simulink model "ultima"  (R2016a)
settings: Solver=ode45  SolverMode=SingleTasking  StartTime=0.0  StopTime=5/60  RelTol=1e-3
libraries: powerlib x98, powerlib_meascontrol x14
settings Model: Creator=hiago  LastModifiedBy=hiago
settings DebuggingCC: SFUnexpectedBacktrackingDiag=error  SFNoUnconditionalDefaultTransitionDiag=error
settings SFSimCC: SimUseLocalCustomCode=on
settings RTWCC: RTWUseLocalCustomCode=on
settings GRTTargetCC: TargetLangStandard=C99 (ISO)  GeneratePreprocessorConditionals=Use local settings
settings ConfigComp: CovMetricSettings=dwe  CovHtmlReporting=off  CovSaveCumulativeToWorkspaceVar=off  CovSaveSingleToWorkspaceVar=off  CovExternalEMLEnable=on

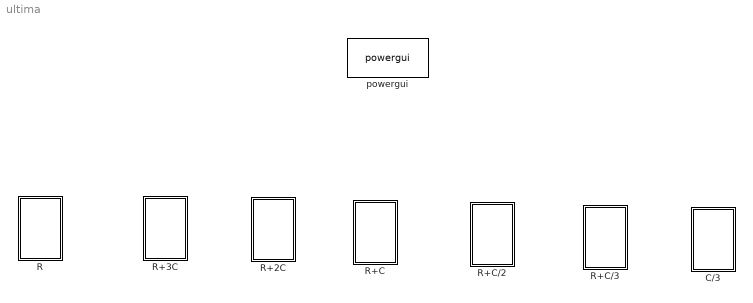
== system ultima ==
  C/3 : Subsystem
  R : Subsystem
  R+2C : Subsystem
  R+3C : Subsystem
  R+C : Subsystem
  R+C/2 : Subsystem
  R+C/3 : Subsystem
  powergui : powerlib/powergui  Priority=1  SimulationMode=Discrete  SampleTime=5e-5  frequency=60  Iterations=50  frequencyindice=60  Pbase=100e6  ErrMax=1e-4  UnitsV=kV  UnitsW=MW  buscounter=0  FunctionMessages=off  echomessages=off  EnableUseOfTLC=off  CurrentSourceSwitches=off  DisableSnubberDevices=off  DisableRonSwitches=off  DisableVfSwitches=off  DisplayEquations=off  SolverType=Tustin/Backward Euler (TBE)  Interpol=off  ExternalGateDelay=off  methode=off  Ts=100  x0status=blocks  SPID=on  SwTol=0  HookPort=off  RestoreLinks=warning  ResistiveCurrentMeasurement=off  Frange=[0:2:500]  Ylog=off  Xlog=on  ShowGrid=off  save=off  variable=ZData  structure=0  ZoomFFT=off  StartTime=0.0  cycles=1  DisplayStyle=1  fundamental=60  FreqAxis=off  MaxFrequency=1000  frequencyindicesteady=1  RmsSteady=1  display=off

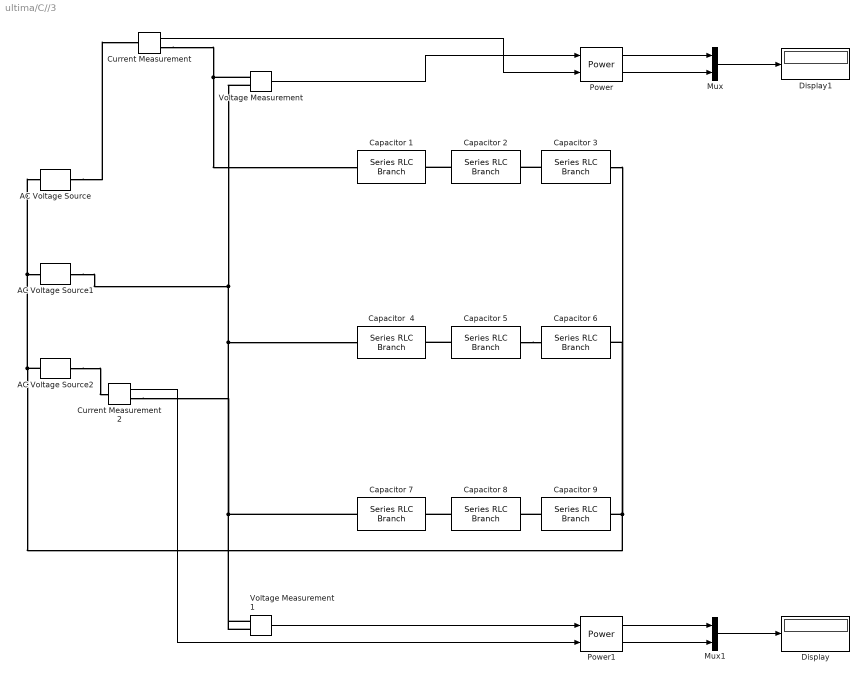
== system ultima/C//3 ==
  AC Voltage Source : powerlib/Electrical Sources/AC Voltage Source  Amplitude=127*sqrt(2)  Phase=0  Frequency=60  SampleTime=5e-5  Measurements=None  BusType=swing  Pref=10e3  Qref=0  Qmin=-inf  Qmax=+inf
  AC Voltage Source1 : powerlib/Electrical Sources/AC Voltage Source  Amplitude=127*sqrt(2)  Phase=-120  Frequency=60  SampleTime=5e-5  Measurements=None  BusType=swing  Pref=10e3  Qref=0  Qmin=-inf  Qmax=+inf
  AC Voltage Source2 : powerlib/Electrical Sources/AC Voltage Source  Amplitude=127*sqrt(2)  Phase=120  Frequency=60  SampleTime=5e-5  Measurements=None  BusType=swing  Pref=10e3  Qref=0  Qmin=-inf  Qmax=+inf
  Capacitor  4 : powerlib/Elements/Series RLC Branch  LConnTagsString=__new0  RConnTagsString=__new0  BranchType=RC  Resistance=1  Inductance=1e-3  SetiL0=off  InitialCurrent=0  Capacitance=22e-6  Setx0=off  InitialVoltage=0  Measurements=None
  "Capacitor 1 " : powerlib/Elements/Series RLC Branch  LConnTagsString=__new0  RConnTagsString=__new0  BranchType=RC  Resistance=1  Inductance=1e-3  SetiL0=off  InitialCurrent=0  Capacitance=22e-6  Setx0=off  InitialVoltage=0  Measurements=None
  Capacitor {2..3,6,8..9} (5 alike) : powerlib/Elements/Series RLC Branch  LConnTagsString=__new0  RConnTagsString=__new0  BranchType=C  Resistance=100  Inductance=1e-3  SetiL0=off  InitialCurrent=0  Capacitance=22e-6  Setx0=off  InitialVoltage=0  Measurements=None
  "Capacitor 5 " : powerlib/Elements/Series RLC Branch  LConnTagsString=__new0  RConnTagsString=__new0  BranchType=C  Resistance=100  Inductance=1e-3  SetiL0=off  InitialCurrent=0  Capacitance=22e-6  Setx0=off  InitialVoltage=0  Measurements=None
  Capacitor 7 : powerlib/Elements/Series RLC Branch  LConnTagsString=__new0  RConnTagsString=__new0  BranchType=RC  Resistance=1  Inductance=1e-3  SetiL0=off  InitialCurrent=0  Capacitance=22e-6  Setx0=off  InitialVoltage=0  Measurements=None
  Current Measurement : powerlib/Measurements/Current Measurement  PhasorSimulation=off  OutputType=Complex  PSBequivalent=0
  Current Measurement2 : powerlib/Measurements/Current Measurement  PhasorSimulation=off  OutputType=Complex  PSBequivalent=0
  Display : Display
  Display1 : Display
  Mux : Mux  Inputs=2
  Mux1 : Mux  Inputs=2
  Power : powerlib_meascontrol/Measurements/Power  Freq=60  Vinit=[1, 0]  Iinit=[1, 0]  Ts=5e-5
  Power1 : powerlib_meascontrol/Measurements/Power  Freq=60  Vinit=[1, 0]  Iinit=[1, 0]  Ts=5e-5
  Voltage Measurement : powerlib/Measurements/Voltage Measurement  PhasorSimulation=off  OutputType=Complex  PSBequivalent=0
  Voltage Measurement1 : powerlib/Measurements/Voltage Measurement  PhasorSimulation=off  OutputType=Complex  PSBequivalent=0
  wires:
  Power1/2 -> Mux1/2
  Power/2 -> Mux/2
  Current Measurement2/1 -> Power1/2
  Current Measurement/1 -> Power/2
  Voltage Measurement/1 -> Power/1
  Power/1 -> Mux/1
  Mux/1 -> Display1/1
  Power1/1 -> Mux1/1
  Voltage Measurement1/1 -> Power1/1
  Mux1/1 -> Display/1
  connections:
  AC Voltage Source2/LConn1 -- Capacitor 6/LConn1 -- Capacitor 3/LConn1 -- Capacitor 9/LConn1 -- AC Voltage Source/LConn1 -- AC Voltage Source1/LConn1
  Voltage Measurement1/LConn1 -- Capacitor 7/RConn1 -- Current Measurement2/RConn1
  AC Voltage Source/RConn1 -- Current Measurement/LConn1
  Current Measurement/RConn1 -- "Capacitor 1 "/RConn1 -- Voltage Measurement/LConn1
  Capacitor 2/RConn1 -- "Capacitor 1 "/LConn1
  AC Voltage Source2/RConn1 -- Current Measurement2/LConn1
  Voltage Measurement1/LConn2 -- Capacitor  4/RConn1 -- AC Voltage Source1/RConn1 -- Voltage Measurement/LConn2
  Capacitor 3/RConn1 -- Capacitor 2/LConn1
  "Capacitor 5 "/RConn1 -- Capacitor  4/LConn1
  "Capacitor 5 "/LConn1 -- Capacitor 6/RConn1
  Capacitor 9/RConn1 -- Capacitor 8/LConn1
  Capacitor 8/RConn1 -- Capacitor 7/LConn1

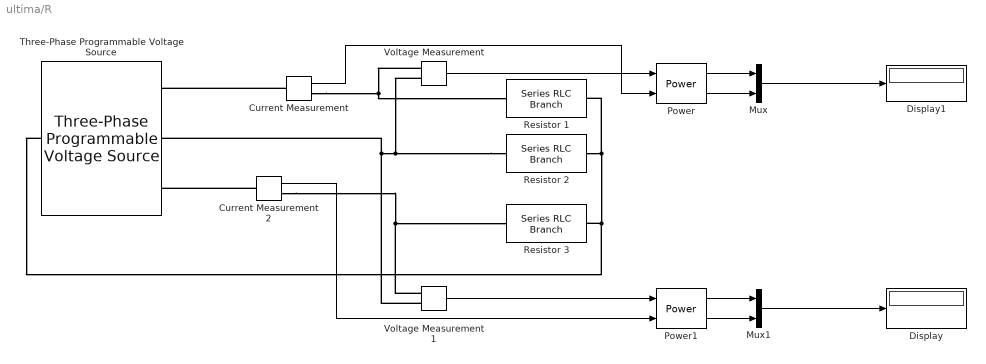
== system ultima/R ==
  Current Measurement : powerlib/Measurements/Current Measurement  PhasorSimulation=off  OutputType=Complex  PSBequivalent=0
  Current Measurement2 : powerlib/Measurements/Current Measurement  PhasorSimulation=off  OutputType=Complex  PSBequivalent=0
  Display : Display
  Display1 : Display
  Mux : Mux  Inputs=2
  Mux1 : Mux  Inputs=2
  Power : powerlib_meascontrol/Measurements/Power  Freq=60  Vinit=[1, 0]  Iinit=[1, 0]  Ts=5e-5
  Power1 : powerlib_meascontrol/Measurements/Power  Freq=60  Vinit=[1, 0]  Iinit=[1, 0]  Ts=5e-5
  Resistor 1 : powerlib/Elements/Series RLC Branch  LConnTagsString=__new0  RConnTagsString=__new0  BranchType=R  Resistance=100  Inductance=1e-3  SetiL0=off  InitialCurrent=0  Capacitance=1e-6  Setx0=off  InitialVoltage=0  Measurements=None
  Resistor 2 : powerlib/Elements/Series RLC Branch  LConnTagsString=__new0  RConnTagsString=__new0  BranchType=R  Resistance=100  Inductance=1e-3  SetiL0=off  InitialCurrent=0  Capacitance=1e-6  Setx0=off  InitialVoltage=0  Measurements=None
  Resistor 3 : powerlib/Elements/Series RLC Branch  LConnTagsString=__new0  RConnTagsString=__new0  BranchType=R  Resistance=100  Inductance=1e-3  SetiL0=off  InitialCurrent=0  Capacitance=1e-6  Setx0=off  InitialVoltage=0  Measurements=None
  Three-Phase Programmable Voltage Source : powerlib/Electrical Sources/Three-Phase Programmable Voltage Source  PositiveSequence="[220  0 60]"  VariationEntity=None  VariationType=Table of time-amplitude pairs  VariationTypeAlt=Step  VariationStep=0.5  VariationRate=10  VariationMagnitude=0.3  VariationFrequency=2  VariationTiming=[1 2]  VariationPhaseA=off  Amplitudes=[1 0.8 1.2 1.0]  TimeValues=[0 0.1 0.15 0.2]  HarmonicGeneration=off  HarmonicA=[3 0.2 -25 0]  HarmonicB=[2 0.15 35 2]  Timing="[0.05  3]"  BusType=swing  Pref=0  Qref=0  Qmin=-inf  Qmax=inf
  Voltage Measurement : powerlib/Measurements/Voltage Measurement  PhasorSimulation=off  OutputType=Complex  PSBequivalent=0
  Voltage Measurement1 : powerlib/Measurements/Voltage Measurement  PhasorSimulation=off  OutputType=Complex  PSBequivalent=0
  wires:
  Mux1/1 -> Display/1
  Voltage Measurement1/1 -> Power1/1
  Voltage Measurement/1 -> Power/1
  Power1/2 -> Mux1/2
  Current Measurement/1 -> Power/2
  Power/1 -> Mux/1
  Mux/1 -> Display1/1
  Power/2 -> Mux/2
  Power1/1 -> Mux1/1
  Current Measurement2/1 -> Power1/2
  connections:
  Voltage Measurement1/LConn1 -- Resistor 3/LConn1 -- Current Measurement2/RConn1
  Current Measurement/RConn1 -- Resistor 1/LConn1 -- Voltage Measurement/LConn1
  Current Measurement/LConn1 -- Three-Phase Programmable Voltage Source/RConn1
  Resistor 2/LConn1 -- Voltage Measurement1/LConn2 -- Three-Phase Programmable Voltage Source/RConn2 -- Voltage Measurement/LConn2
  Resistor 2/RConn1 -- Three-Phase Programmable Voltage Source/LConn1 -- Resistor 3/RConn1 -- Resistor 1/RConn1
  Current Measurement2/LConn1 -- Three-Phase Programmable Voltage Source/RConn3

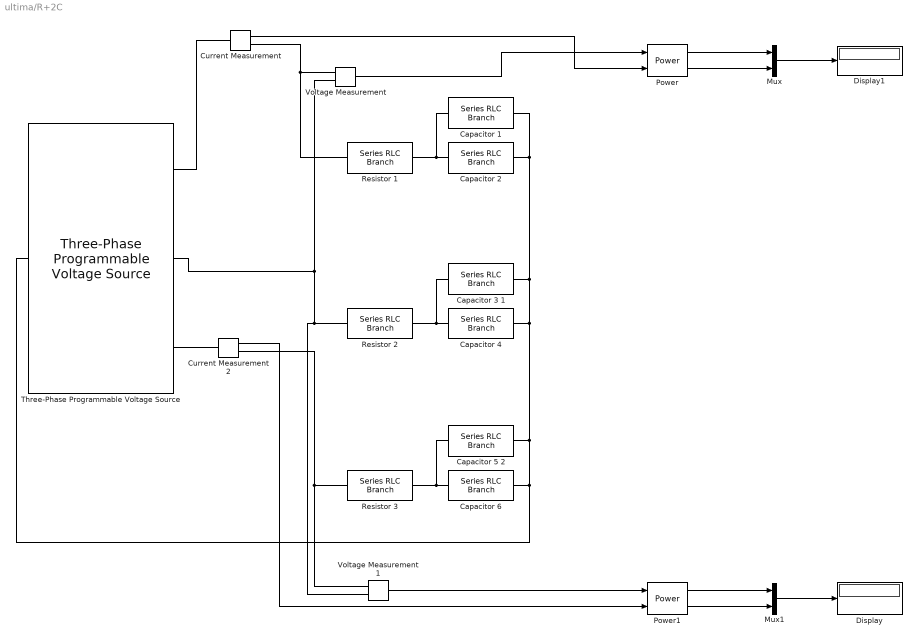
== system ultima/R+2C ==
  "Capacitor 1 " : powerlib/Elements/Series RLC Branch  LConnTagsString=__new0  RConnTagsString=__new0  BranchType=C  Resistance=100  Inductance=1e-3  SetiL0=off  InitialCurrent=0  Capacitance=22e-6  Setx0=off  InitialVoltage=0  Measurements=None
  Capacitor 2 : powerlib/Elements/Series RLC Branch  LConnTagsString=__new0  RConnTagsString=__new0  BranchType=C  Resistance=100  Inductance=1e-3  SetiL0=off  InitialCurrent=0  Capacitance=22e-6  Setx0=off  InitialVoltage=0  Measurements=None
  Capacitor 3 1 : powerlib/Elements/Series RLC Branch  LConnTagsString=__new0  RConnTagsString=__new0  BranchType=C  Resistance=100  Inductance=1e-3  SetiL0=off  InitialCurrent=0  Capacitance=22e-6  Setx0=off  InitialVoltage=0  Measurements=None
  Capacitor 4 : powerlib/Elements/Series RLC Branch  LConnTagsString=__new0  RConnTagsString=__new0  BranchType=C  Resistance=100  Inductance=1e-3  SetiL0=off  InitialCurrent=0  Capacitance=22e-6  Setx0=off  InitialVoltage=0  Measurements=None
  Capacitor 5 2 : powerlib/Elements/Series RLC Branch  LConnTagsString=__new0  RConnTagsString=__new0  BranchType=C  Resistance=100  Inductance=1e-3  SetiL0=off  InitialCurrent=0  Capacitance=22e-6  Setx0=off  InitialVoltage=0  Measurements=None
  Capacitor 6 : powerlib/Elements/Series RLC Branch  LConnTagsString=__new0  RConnTagsString=__new0  BranchType=C  Resistance=100  Inductance=1e-3  SetiL0=off  InitialCurrent=0  Capacitance=22e-6  Setx0=off  InitialVoltage=0  Measurements=None
  Current Measurement : powerlib/Measurements/Current Measurement  PhasorSimulation=off  OutputType=Complex  PSBequivalent=0
  Current Measurement2 : powerlib/Measurements/Current Measurement  PhasorSimulation=off  OutputType=Complex  PSBequivalent=0
  Display : Display
  Display1 : Display
  Mux : Mux  Inputs=2
  Mux1 : Mux  Inputs=2
  Power : powerlib_meascontrol/Measurements/Power  Freq=60  Vinit=[1, 0]  Iinit=[1, 0]  Ts=5e-5
  Power1 : powerlib_meascontrol/Measurements/Power  Freq=60  Vinit=[1, 0]  Iinit=[1, 0]  Ts=5e-5
  Resistor 1 : powerlib/Elements/Series RLC Branch  LConnTagsString=__new0  RConnTagsString=__new0  BranchType=R  Resistance=100  Inductance=1e-3  SetiL0=off  InitialCurrent=0  Capacitance=1e-6  Setx0=off  InitialVoltage=0  Measurements=None
  Resistor 2 : powerlib/Elements/Series RLC Branch  LConnTagsString=__new0  RConnTagsString=__new0  BranchType=R  Resistance=100  Inductance=1e-3  SetiL0=off  InitialCurrent=0  Capacitance=1e-6  Setx0=off  InitialVoltage=0  Measurements=None
  Resistor 3 : powerlib/Elements/Series RLC Branch  LConnTagsString=__new0  RConnTagsString=__new0  BranchType=R  Resistance=100  Inductance=1e-3  SetiL0=off  InitialCurrent=0  Capacitance=1e-6  Setx0=off  InitialVoltage=0  Measurements=None
  Three-Phase Programmable Voltage Source : powerlib/Electrical Sources/Three-Phase Programmable Voltage Source  PositiveSequence="[220  0 60]"  VariationEntity=None  VariationType=Table of time-amplitude pairs  VariationTypeAlt=Step  VariationStep=0.5  VariationRate=10  VariationMagnitude=0.3  VariationFrequency=2  VariationTiming=[1 2]  VariationPhaseA=off  Amplitudes=[1 0.8 1.2 1.0]  TimeValues=[0 0.1 0.15 0.2]  HarmonicGeneration=off  HarmonicA=[3 0.2 -25 0]  HarmonicB=[2 0.15 35 2]  Timing="[0.05  3]"  BusType=swing  Pref=0  Qref=0  Qmin=-inf  Qmax=inf
  Voltage Measurement : powerlib/Measurements/Voltage Measurement  PhasorSimulation=off  OutputType=Complex  PSBequivalent=0
  Voltage Measurement1 : powerlib/Measurements/Voltage Measurement  PhasorSimulation=off  OutputType=Complex  PSBequivalent=0
  wires:
  Voltage Measurement1/1 -> Power1/1
  Power1/2 -> Mux1/2
  Power/1 -> Mux/1
  Power1/1 -> Mux1/1
  Mux1/1 -> Display/1
  Current Measurement2/1 -> Power1/2
  Power/2 -> Mux/2
  Voltage Measurement/1 -> Power/1
  Current Measurement/1 -> Power/2
  Mux/1 -> Display1/1
  connections:
  Resistor 3/LConn1 -- Current Measurement2/RConn1 -- Voltage Measurement1/LConn1
  Current Measurement/RConn1 -- Resistor 1/LConn1 -- Voltage Measurement/LConn1
  Voltage Measurement/LConn2 -- Voltage Measurement1/LConn2 -- Resistor 2/LConn1 -- Three-Phase Programmable Voltage Source/RConn2
  Current Measurement/LConn1 -- Three-Phase Programmable Voltage Source/RConn1
  Current Measurement2/LConn1 -- Three-Phase Programmable Voltage Source/RConn3
  Capacitor 6/RConn1 -- Three-Phase Programmable Voltage Source/LConn1 -- Capacitor 5 2/RConn1 -- Capacitor 4/RConn1 -- Capacitor 3 1/RConn1 -- Capacitor 2/RConn1 -- "Capacitor 1 "/RConn1
  Capacitor 5 2/LConn1 -- Resistor 3/RConn1 -- Capacitor 6/LConn1
  Capacitor 4/LConn1 -- Resistor 2/RConn1 -- Capacitor 3 1/LConn1
  Capacitor 2/LConn1 -- Resistor 1/RConn1 -- "Capacitor 1 "/LConn1

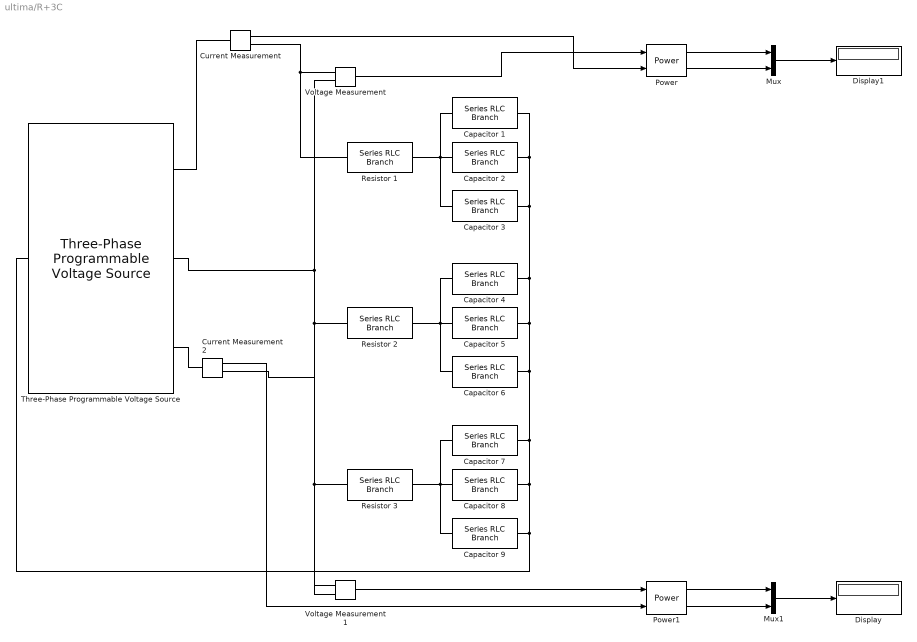
== system ultima/R+3C ==
  Capacitor {1..9} (9 alike) : powerlib/Elements/Series RLC Branch  LConnTagsString=__new0  RConnTagsString=__new0  BranchType=C  Resistance=100  Inductance=1e-3  SetiL0=off  InitialCurrent=0  Capacitance=22e-6  Setx0=off  InitialVoltage=0  Measurements=None
  Current Measurement : powerlib/Measurements/Current Measurement  PhasorSimulation=off  OutputType=Complex  PSBequivalent=0
  Current Measurement2 : powerlib/Measurements/Current Measurement  PhasorSimulation=off  OutputType=Complex  PSBequivalent=0
  Display : Display
  Display1 : Display
  Mux : Mux  Inputs=2
  Mux1 : Mux  Inputs=2
  Power : powerlib_meascontrol/Measurements/Power  Freq=60  Vinit=[1, 0]  Iinit=[1, 0]  Ts=5e-5
  Power1 : powerlib_meascontrol/Measurements/Power  Freq=60  Vinit=[1, 0]  Iinit=[1, 0]  Ts=5e-5
  Resistor 1 : powerlib/Elements/Series RLC Branch  LConnTagsString=__new0  RConnTagsString=__new0  BranchType=R  Resistance=100  Inductance=1e-3  SetiL0=off  InitialCurrent=0  Capacitance=1e-6  Setx0=off  InitialVoltage=0  Measurements=None
  Resistor 2 : powerlib/Elements/Series RLC Branch  LConnTagsString=__new0  RConnTagsString=__new0  BranchType=R  Resistance=100  Inductance=1e-3  SetiL0=off  InitialCurrent=0  Capacitance=1e-6  Setx0=off  InitialVoltage=0  Measurements=None
  Resistor 3 : powerlib/Elements/Series RLC Branch  LConnTagsString=__new0  RConnTagsString=__new0  BranchType=R  Resistance=100  Inductance=1e-3  SetiL0=off  InitialCurrent=0  Capacitance=1e-6  Setx0=off  InitialVoltage=0  Measurements=None
  Three-Phase Programmable Voltage Source : powerlib/Electrical Sources/Three-Phase Programmable Voltage Source  PositiveSequence="[220  0 60]"  VariationEntity=None  VariationType=Table of time-amplitude pairs  VariationTypeAlt=Step  VariationStep=0.5  VariationRate=10  VariationMagnitude=0.3  VariationFrequency=2  VariationTiming=[1 2]  VariationPhaseA=off  Amplitudes=[1 0.8 1.2 1.0]  TimeValues=[0 0.1 0.15 0.2]  HarmonicGeneration=off  HarmonicA=[3 0.2 -25 0]  HarmonicB=[2 0.15 35 2]  Timing="[0.05  3]"  BusType=swing  Pref=0  Qref=0  Qmin=-inf  Qmax=inf
  Voltage Measurement : powerlib/Measurements/Voltage Measurement  PhasorSimulation=off  OutputType=Complex  PSBequivalent=0
  Voltage Measurement1 : powerlib/Measurements/Voltage Measurement  PhasorSimulation=off  OutputType=Complex  PSBequivalent=0
  wires:
  Current Measurement/1 -> Power/2
  Power1/1 -> Mux1/1
  Current Measurement2/1 -> Power1/2
  Power/1 -> Mux/1
  Voltage Measurement/1 -> Power/1
  Mux/1 -> Display1/1
  Power/2 -> Mux/2
  Mux1/1 -> Display/1
  Voltage Measurement1/1 -> Power1/1
  Power1/2 -> Mux1/2
  connections:
  Current Measurement2/LConn1 -- Three-Phase Programmable Voltage Source/RConn3
  Current Measurement2/RConn1 -- Voltage Measurement1/LConn1 -- Resistor 3/LConn1
  Current Measurement/RConn1 -- Resistor 1/LConn1 -- Voltage Measurement/LConn1
  Resistor 2/LConn1 -- Three-Phase Programmable Voltage Source/RConn2 -- Voltage Measurement/LConn2 -- Voltage Measurement1/LConn2
  Current Measurement/LConn1 -- Three-Phase Programmable Voltage Source/RConn1
  Capacitor 3/LConn1 -- Capacitor 1/LConn1 -- Resistor 1/RConn1 -- Capacitor 2/LConn1
  Capacitor 8/RConn1 -- Three-Phase Programmable Voltage Source/LConn1 -- Capacitor 9/RConn1 -- Capacitor 5/RConn1 -- Capacitor 1/RConn1 -- Capacitor 2/RConn1 -- Capacitor 3/RConn1 -- Capacitor 4/RConn1 -- Capacitor 6/RConn1 -- Capacitor 7/RConn1
  Resistor 2/RConn1 -- Capacitor 6/LConn1 -- Capacitor 4/LConn1 -- Capacitor 5/LConn1
  Capacitor 8/LConn1 -- Capacitor 9/LConn1 -- Resistor 3/RConn1 -- Capacitor 7/LConn1

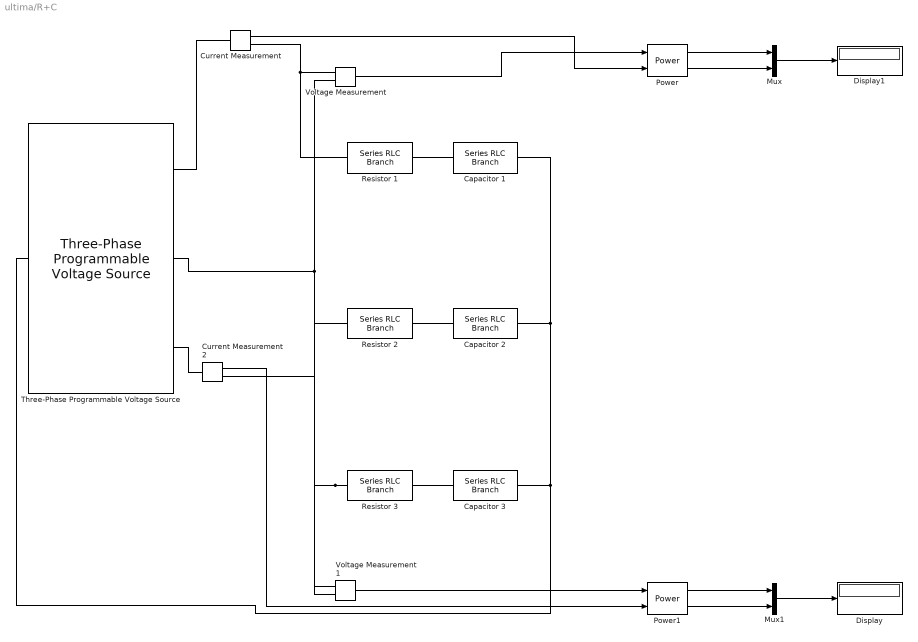
== system ultima/R+C ==
  Capacitor 1 : powerlib/Elements/Series RLC Branch  LConnTagsString=__new0  RConnTagsString=__new0  BranchType=C  Resistance=100  Inductance=1e-3  SetiL0=off  InitialCurrent=0  Capacitance=22e-6  Setx0=off  InitialVoltage=0  Measurements=None
  Capacitor 2 : powerlib/Elements/Series RLC Branch  LConnTagsString=__new0  RConnTagsString=__new0  BranchType=C  Resistance=100  Inductance=1e-3  SetiL0=off  InitialCurrent=0  Capacitance=22e-6  Setx0=off  InitialVoltage=0  Measurements=None
  Capacitor 3 : powerlib/Elements/Series RLC Branch  LConnTagsString=__new0  RConnTagsString=__new0  BranchType=C  Resistance=100  Inductance=1e-3  SetiL0=off  InitialCurrent=0  Capacitance=22e-6  Setx0=off  InitialVoltage=0  Measurements=None
  Current Measurement : powerlib/Measurements/Current Measurement  PhasorSimulation=off  OutputType=Complex  PSBequivalent=0
  Current Measurement2 : powerlib/Measurements/Current Measurement  PhasorSimulation=off  OutputType=Complex  PSBequivalent=0
  Display : Display
  Display1 : Display
  Mux : Mux  Inputs=2
  Mux1 : Mux  Inputs=2
  Power : powerlib_meascontrol/Measurements/Power  Freq=60  Vinit=[1, 0]  Iinit=[1, 0]  Ts=5e-5
  Power1 : powerlib_meascontrol/Measurements/Power  Freq=60  Vinit=[1, 0]  Iinit=[1, 0]  Ts=5e-5
  Resistor 1 : powerlib/Elements/Series RLC Branch  LConnTagsString=__new0  RConnTagsString=__new0  BranchType=R  Resistance=100  Inductance=1e-3  SetiL0=off  InitialCurrent=0  Capacitance=1e-6  Setx0=off  InitialVoltage=0  Measurements=None
  Resistor 2 : powerlib/Elements/Series RLC Branch  LConnTagsString=__new0  RConnTagsString=__new0  BranchType=R  Resistance=100  Inductance=1e-3  SetiL0=off  InitialCurrent=0  Capacitance=1e-6  Setx0=off  InitialVoltage=0  Measurements=None
  Resistor 3 : powerlib/Elements/Series RLC Branch  LConnTagsString=__new0  RConnTagsString=__new0  BranchType=R  Resistance=100  Inductance=1e-3  SetiL0=off  InitialCurrent=0  Capacitance=1e-6  Setx0=off  InitialVoltage=0  Measurements=None
  Three-Phase Programmable Voltage Source : powerlib/Electrical Sources/Three-Phase Programmable Voltage Source  PositiveSequence="[220  0 60]"  VariationEntity=None  VariationType=Table of time-amplitude pairs  VariationTypeAlt=Step  VariationStep=0.5  VariationRate=10  VariationMagnitude=0.3  VariationFrequency=2  VariationTiming=[1 2]  VariationPhaseA=off  Amplitudes=[1 0.8 1.2 1.0]  TimeValues=[0 0.1 0.15 0.2]  HarmonicGeneration=off  HarmonicA=[3 0.2 -25 0]  HarmonicB=[2 0.15 35 2]  Timing="[0.05  3]"  BusType=swing  Pref=0  Qref=0  Qmin=-inf  Qmax=inf
  Voltage Measurement : powerlib/Measurements/Voltage Measurement  PhasorSimulation=off  OutputType=Complex  PSBequivalent=0
  Voltage Measurement1 : powerlib/Measurements/Voltage Measurement  PhasorSimulation=off  OutputType=Complex  PSBequivalent=0
  wires:
  Current Measurement/1 -> Power/2
  Mux1/1 -> Display/1
  Current Measurement2/1 -> Power1/2
  Voltage Measurement/1 -> Power/1
  Mux/1 -> Display1/1
  Power/2 -> Mux/2
  Power1/1 -> Mux1/1
  Power/1 -> Mux/1
  Power1/2 -> Mux1/2
  Voltage Measurement1/1 -> Power1/1
  connections:
  Three-Phase Programmable Voltage Source/LConn1 -- Capacitor 3/RConn1 -- Capacitor 1/RConn1 -- Capacitor 2/RConn1
  Voltage Measurement/LConn2 -- Three-Phase Programmable Voltage Source/RConn2 -- Voltage Measurement1/LConn2 -- Resistor 2/LConn1
  Resistor 3/LConn1 -- Current Measurement2/RConn1 -- Voltage Measurement1/LConn1
  Current Measurement/RConn1 -- Resistor 1/LConn1 -- Voltage Measurement/LConn1
  Current Measurement/LConn1 -- Three-Phase Programmable Voltage Source/RConn1
  Current Measurement2/LConn1 -- Three-Phase Programmable Voltage Source/RConn3
  Resistor 1/RConn1 -- Capacitor 1/LConn1
  Resistor 3/RConn1 -- Capacitor 3/LConn1
  Capacitor 2/LConn1 -- Resistor 2/RConn1

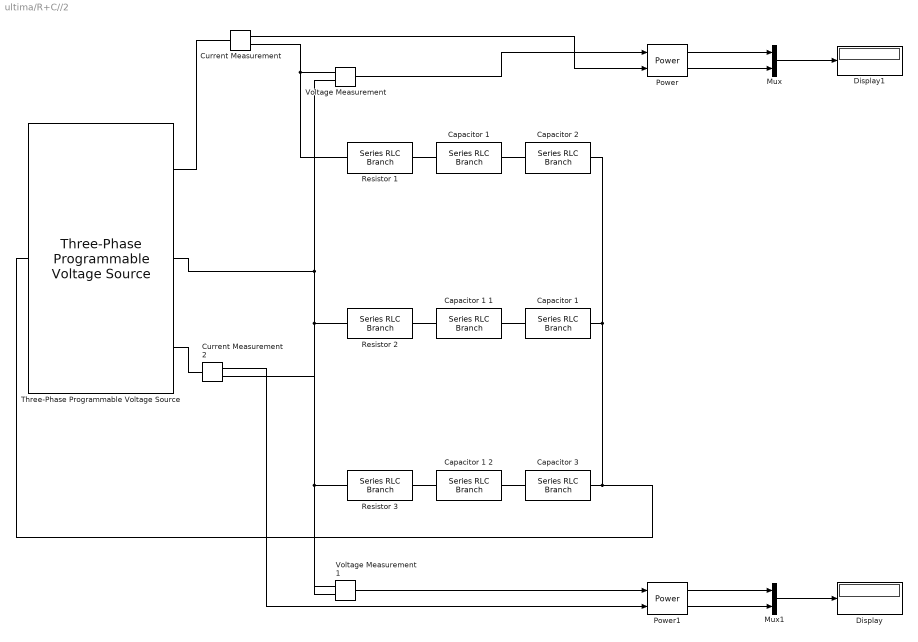
== system ultima/R+C//2 ==
  Capacitor 1 : powerlib/Elements/Series RLC Branch  LConnTagsString=__new0  RConnTagsString=__new0  BranchType=C  Resistance=100  Inductance=1e-3  SetiL0=off  InitialCurrent=0  Capacitance=22e-6  Setx0=off  InitialVoltage=0  Measurements=None
  "Capacitor 1 " : powerlib/Elements/Series RLC Branch  LConnTagsString=__new0  RConnTagsString=__new0  BranchType=C  Resistance=100  Inductance=1e-3  SetiL0=off  InitialCurrent=0  Capacitance=22e-6  Setx0=off  InitialVoltage=0  Measurements=None
  Capacitor 1 1 : powerlib/Elements/Series RLC Branch  LConnTagsString=__new0  RConnTagsString=__new0  BranchType=C  Resistance=100  Inductance=1e-3  SetiL0=off  InitialCurrent=0  Capacitance=22e-6  Setx0=off  InitialVoltage=0  Measurements=None
  Capacitor 1 2 : powerlib/Elements/Series RLC Branch  LConnTagsString=__new0  RConnTagsString=__new0  BranchType=C  Resistance=100  Inductance=1e-3  SetiL0=off  InitialCurrent=0  Capacitance=22e-6  Setx0=off  InitialVoltage=0  Measurements=None
  Capacitor 2 : powerlib/Elements/Series RLC Branch  LConnTagsString=__new0  RConnTagsString=__new0  BranchType=C  Resistance=100  Inductance=1e-3  SetiL0=off  InitialCurrent=0  Capacitance=22e-6  Setx0=off  InitialVoltage=0  Measurements=None
  Capacitor 3 : powerlib/Elements/Series RLC Branch  LConnTagsString=__new0  RConnTagsString=__new0  BranchType=C  Resistance=100  Inductance=1e-3  SetiL0=off  InitialCurrent=0  Capacitance=22e-6  Setx0=off  InitialVoltage=0  Measurements=None
  Current Measurement : powerlib/Measurements/Current Measurement  PhasorSimulation=off  OutputType=Complex  PSBequivalent=0
  Current Measurement2 : powerlib/Measurements/Current Measurement  PhasorSimulation=off  OutputType=Complex  PSBequivalent=0
  Display : Display
  Display1 : Display
  Mux : Mux  Inputs=2
  Mux1 : Mux  Inputs=2
  Power : powerlib_meascontrol/Measurements/Power  Freq=60  Vinit=[1, 0]  Iinit=[1, 0]  Ts=5e-5
  Power1 : powerlib_meascontrol/Measurements/Power  Freq=60  Vinit=[1, 0]  Iinit=[1, 0]  Ts=5e-5
  Resistor 1 : powerlib/Elements/Series RLC Branch  LConnTagsString=__new0  RConnTagsString=__new0  BranchType=R  Resistance=100  Inductance=1e-3  SetiL0=off  InitialCurrent=0  Capacitance=1e-6  Setx0=off  InitialVoltage=0  Measurements=None
  Resistor 2 : powerlib/Elements/Series RLC Branch  LConnTagsString=__new0  RConnTagsString=__new0  BranchType=R  Resistance=100  Inductance=1e-3  SetiL0=off  InitialCurrent=0  Capacitance=1e-6  Setx0=off  InitialVoltage=0  Measurements=None
  Resistor 3 : powerlib/Elements/Series RLC Branch  LConnTagsString=__new0  RConnTagsString=__new0  BranchType=R  Resistance=100  Inductance=1e-3  SetiL0=off  InitialCurrent=0  Capacitance=1e-6  Setx0=off  InitialVoltage=0  Measurements=None
  Three-Phase Programmable Voltage Source : powerlib/Electrical Sources/Three-Phase Programmable Voltage Source  PositiveSequence="[220  0 60]"  VariationEntity=None  VariationType=Table of time-amplitude pairs  VariationTypeAlt=Step  VariationStep=0.5  VariationRate=10  VariationMagnitude=0.3  VariationFrequency=2  VariationTiming=[1 2]  VariationPhaseA=off  Amplitudes=[1 0.8 1.2 1.0]  TimeValues=[0 0.1 0.15 0.2]  HarmonicGeneration=off  HarmonicA=[3 0.2 -25 0]  HarmonicB=[2 0.15 35 2]  Timing="[0.05  3]"  BusType=swing  Pref=0  Qref=0  Qmin=-inf  Qmax=inf
  Voltage Measurement : powerlib/Measurements/Voltage Measurement  PhasorSimulation=off  OutputType=Complex  PSBequivalent=0
  Voltage Measurement1 : powerlib/Measurements/Voltage Measurement  PhasorSimulation=off  OutputType=Complex  PSBequivalent=0
  wires:
  Current Measurement/1 -> Power/2
  Power/1 -> Mux/1
  Current Measurement2/1 -> Power1/2
  Power/2 -> Mux/2
  Voltage Measurement1/1 -> Power1/1
  Voltage Measurement/1 -> Power/1
  Mux1/1 -> Display/1
  Power1/2 -> Mux1/2
  Power1/1 -> Mux1/1
  Mux/1 -> Display1/1
  connections:
  Current Measurement/LConn1 -- Three-Phase Programmable Voltage Source/RConn1
  Current Measurement2/LConn1 -- Three-Phase Programmable Voltage Source/RConn3
  Resistor 2/LConn1 -- Voltage Measurement1/LConn2 -- Three-Phase Programmable Voltage Source/RConn2 -- Voltage Measurement/LConn2
  Resistor 3/LConn1 -- Current Measurement2/RConn1 -- Voltage Measurement1/LConn1
  Current Measurement/RConn1 -- Resistor 1/LConn1 -- Voltage Measurement/LConn1
  "Capacitor 1 "/RConn1 -- Resistor 1/RConn1
  Capacitor 2/RConn1 -- "Capacitor 1 "/LConn1
  Capacitor 1/RConn1 -- Capacitor 1 1/LConn1
  Resistor 2/RConn1 -- Capacitor 1 1/RConn1
  Capacitor 3/RConn1 -- Capacitor 1 2/LConn1
  Capacitor 1 2/RConn1 -- Resistor 3/RConn1
  Three-Phase Programmable Voltage Source/LConn1 -- Capacitor 2/LConn1 -- Capacitor 1/LConn1 -- Capacitor 3/LConn1

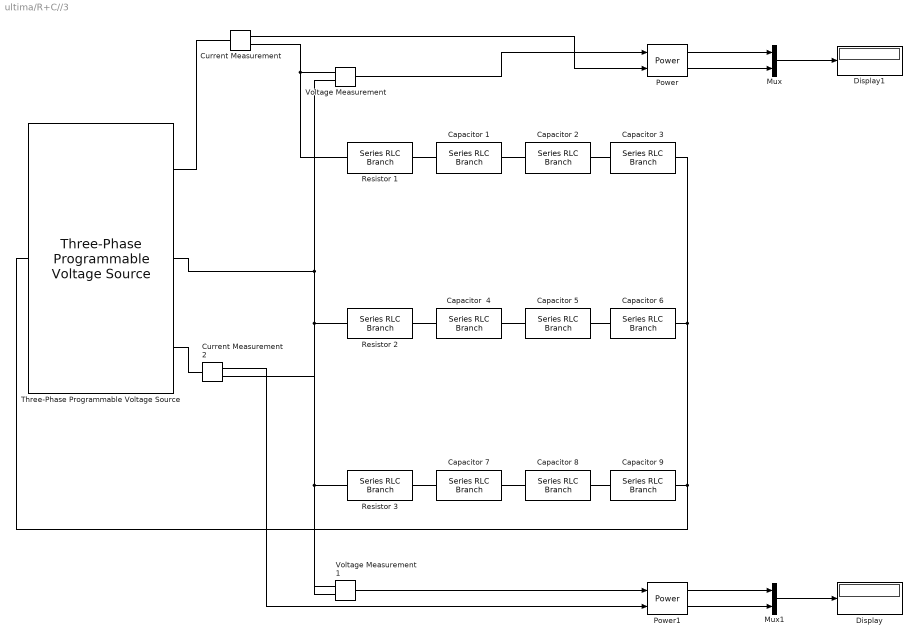
== system ultima/R+C//3 ==
  Capacitor  4 : powerlib/Elements/Series RLC Branch  LConnTagsString=__new0  RConnTagsString=__new0  BranchType=C  Resistance=100  Inductance=1e-3  SetiL0=off  InitialCurrent=0  Capacitance=22e-6  Setx0=off  InitialVoltage=0  Measurements=None
  "Capacitor 1 " : powerlib/Elements/Series RLC Branch  LConnTagsString=__new0  RConnTagsString=__new0  BranchType=C  Resistance=100  Inductance=1e-3  SetiL0=off  InitialCurrent=0  Capacitance=22e-6  Setx0=off  InitialVoltage=0  Measurements=None
  Capacitor {2..3,6..9} (6 alike) : powerlib/Elements/Series RLC Branch  LConnTagsString=__new0  RConnTagsString=__new0  BranchType=C  Resistance=100  Inductance=1e-3  SetiL0=off  InitialCurrent=0  Capacitance=22e-6  Setx0=off  InitialVoltage=0  Measurements=None
  "Capacitor 5 " : powerlib/Elements/Series RLC Branch  LConnTagsString=__new0  RConnTagsString=__new0  BranchType=C  Resistance=100  Inductance=1e-3  SetiL0=off  InitialCurrent=0  Capacitance=22e-6  Setx0=off  InitialVoltage=0  Measurements=None
  Current Measurement : powerlib/Measurements/Current Measurement  PhasorSimulation=off  OutputType=Complex  PSBequivalent=0
  Current Measurement2 : powerlib/Measurements/Current Measurement  PhasorSimulation=off  OutputType=Complex  PSBequivalent=0
  Display : Display
  Display1 : Display
  Mux : Mux  Inputs=2
  Mux1 : Mux  Inputs=2
  Power : powerlib_meascontrol/Measurements/Power  Freq=60  Vinit=[1, 0]  Iinit=[1, 0]  Ts=5e-5
  Power1 : powerlib_meascontrol/Measurements/Power  Freq=60  Vinit=[1, 0]  Iinit=[1, 0]  Ts=5e-5
  Resistor 1 : powerlib/Elements/Series RLC Branch  LConnTagsString=__new0  RConnTagsString=__new0  BranchType=R  Resistance=100  Inductance=1e-3  SetiL0=off  InitialCurrent=0  Capacitance=1e-6  Setx0=off  InitialVoltage=0  Measurements=None
  Resistor 2 : powerlib/Elements/Series RLC Branch  LConnTagsString=__new0  RConnTagsString=__new0  BranchType=R  Resistance=100  Inductance=1e-3  SetiL0=off  InitialCurrent=0  Capacitance=1e-6  Setx0=off  InitialVoltage=0  Measurements=None
  Resistor 3 : powerlib/Elements/Series RLC Branch  LConnTagsString=__new0  RConnTagsString=__new0  BranchType=R  Resistance=100  Inductance=1e-3  SetiL0=off  InitialCurrent=0  Capacitance=1e-6  Setx0=off  InitialVoltage=0  Measurements=None
  Three-Phase Programmable Voltage Source : powerlib/Electrical Sources/Three-Phase Programmable Voltage Source  PositiveSequence="[220  0 60]"  VariationEntity=None  VariationType=Table of time-amplitude pairs  VariationTypeAlt=Step  VariationStep=0.5  VariationRate=10  VariationMagnitude=0.3  VariationFrequency=2  VariationTiming=[1 2]  VariationPhaseA=off  Amplitudes=[1 0.8 1.2 1.0]  TimeValues=[0 0.1 0.15 0.2]  HarmonicGeneration=off  HarmonicA=[3 0.2 -25 0]  HarmonicB=[2 0.15 35 2]  Timing="[0.05  3]"  BusType=swing  Pref=0  Qref=0  Qmin=-inf  Qmax=inf
  Voltage Measurement : powerlib/Measurements/Voltage Measurement  PhasorSimulation=off  OutputType=Complex  PSBequivalent=0
  Voltage Measurement1 : powerlib/Measurements/Voltage Measurement  PhasorSimulation=off  OutputType=Complex  PSBequivalent=0
  wires:
  Voltage Measurement/1 -> Power/1
  Power/2 -> Mux/2
  Mux1/1 -> Display/1
  Current Measurement/1 -> Power/2
  Power1/2 -> Mux1/2
  Power1/1 -> Mux1/1
  Voltage Measurement1/1 -> Power1/1
  Power/1 -> Mux/1
  Current Measurement2/1 -> Power1/2
  Mux/1 -> Display1/1
  connections:
  Voltage Measurement/LConn2 -- Three-Phase Programmable Voltage Source/RConn2 -- Voltage Measurement1/LConn2 -- Resistor 2/LConn1
  Current Measurement/RConn1 -- Resistor 1/LConn1 -- Voltage Measurement/LConn1
  "Capacitor 1 "/RConn1 -- Resistor 1/RConn1
  Capacitor 8/RConn1 -- Capacitor 7/LConn1
  Resistor 3/LConn1 -- Current Measurement2/RConn1 -- Voltage Measurement1/LConn1
  Capacitor 7/RConn1 -- Resistor 3/RConn1
  "Capacitor 5 "/RConn1 -- Capacitor  4/LConn1
  Current Measurement/LConn1 -- Three-Phase Programmable Voltage Source/RConn1
  Resistor 2/RConn1 -- Capacitor  4/RConn1
  Capacitor 2/RConn1 -- "Capacitor 1 "/LConn1
  Current Measurement2/LConn1 -- Three-Phase Programmable Voltage Source/RConn3
  Capacitor 3/RConn1 -- Capacitor 2/LConn1
  Capacitor 9/RConn1 -- Capacitor 8/LConn1
  "Capacitor 5 "/LConn1 -- Capacitor 6/RConn1
  Capacitor 3/LConn1 -- Three-Phase Programmable Voltage Source/LConn1 -- Capacitor 9/LConn1 -- Capacitor 6/LConn1
